simulink model "multiTask"  (R2015b)
settings: Solver=FixedStepDiscrete  SolverMode=MultiTasking  StartTime=0.0  StopTime=inf  FixedStep=1/10  RelTol=1e-3
undefined symbols (not defined in the file): Green, led0
libraries: simulink x1, embdlinuxlib x1
settings Model: SimulationMode=external  ExtModeEnableFloating=off  ExtModeTrigDuration=100  Creator=Nik Descher  LastModifiedBy=Nik Descher
settings DataIOCC: LimitDataPoints=off
settings OptimizationCC: OptimizeModelRefInitCode=on  LifeSpan=1
settings HardwareCC: ProdBitPerPointer=32  ProdLargestAtomicInteger=Long  ProdLargestAtomicFloat=Double  ProdWordSize=32  ProdHWDeviceType=ARM Compatible->ARM Cortex
settings RTWCC: SystemTargetFile=realtime.tlc  GenerateMakefile=off  TemplateMakefile=realtime.tmf  Description=Run on Target Hardware  RTWVerbose=off
settings STFCustomTargetCC: TargetLibSuffix=.a  GenerateSampleERTMain=on  ConcurrentExecutionCompliant=off  GeneratePreprocessorConditionals=Use local settings  ERTCustomFileBanners=on  SupportNonInlinedSFcns=off  SupportVariableSizeSignals=on  MATLABClassNameForMDSCustomization=Simulink.SoftwareTarget.ERTCustomization  CPPClassGenCompliant=off  GRTInterface=off  SystemTargetFile=realtime.tlc
settings ERTTargetCC: GenerateSampleERTMain=on  ParMdlRefBuildCompliant=off  CompOptLevelCompliant=off  ConcurrentExecutionCompliant=off  CombineOutputUpdateFcns=off  ERTFirstTimeCompliant=off  SupportContinuousTime=on  SupportVariableSizeSignals=on  ModelStepFunctionPrototypeControlCompliant=off  CPPClassGenCompliant=off  UseToolchainInfoCompliant=off  ExtModeMexArgs='192.168.1.248' 0 17725  ERTSrcFileBannerTemplate=realtime_code_template.cgt  ERTHdrFileBannerTemplate=realtime_code_template.cgt  ERTDataSrcFileTemplate=realtime_code_template.cgt  ERTDataHdrFileTemplate=realtime_code_template.cgt  ERTCustomFileTemplate=realtime_file_process.tlc

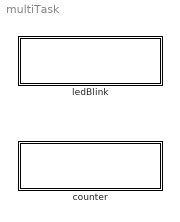
== system multiTask ==
  counter : Subsystem  TreatAsAtomicUnit=on  SystemSampleTime=1
  ledBlink : Subsystem  TreatAsAtomicUnit=on  SystemSampleTime=1/10

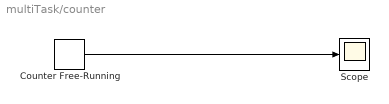
== system multiTask/counter ==
  Counter Free-Running : simulink/Sources/Counter Free-Running  NumBits=32  tsamp=-1
  Scope : Scope
  wires:
  Counter Free-Running/1 -> Scope/1

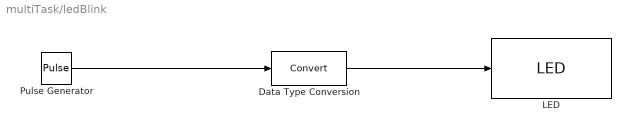
== system multiTask/ledBlink ==
  Data Type Conversion : DataTypeConversion
  LED : embdlinuxlib/LED  board=Pi 2 Model B  led=led0 (Green)  blockPlatform=Raspberry Pi
  Pulse Generator : DiscretePulseGenerator  PulseType=Time based  PulseWidth=50
  wires:
  Data Type Conversion/1 -> LED/1
  Pulse Generator/1 -> Data Type Conversion/1
